simulink model "online_ups"  (R2024b)
settings: Solver=VariableStepAuto  StartTime=0.0  StopTime=0.2  RelTol=1e-3
libraries: spsIGBTDiodeLib x4, spsCurrentMeasurementLib x2, spsVoltageMeasurementLib x2, spsDCVoltageSourceLib x1, spsTriangleGeneratorLib x1, spsSeriesRLCBranchLib x1, sps_lib x1
settings Model: Creator=rushi  LastModifiedBy=rushi
settings DataIOCC: ReturnWorkspaceOutputs=off

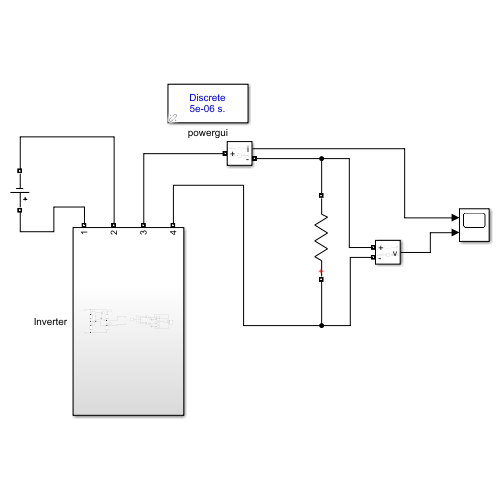
[thumbnail: Simulink's stored preview of the top-level diagram]
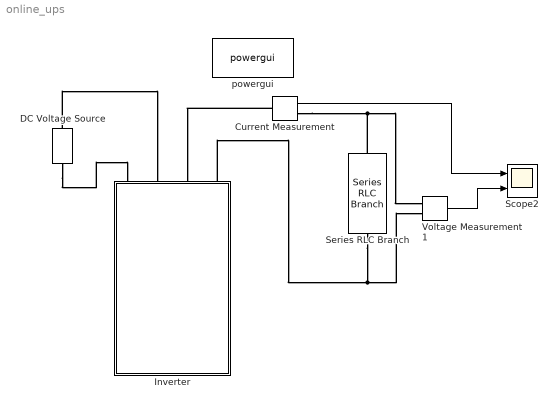
== system online_ups ==
  Current Measurement : spsCurrentMeasurementLib/Current Measurement  PhasorSimulation=off  OutputType=Complex  PSBequivalent=0
  DC Voltage Source : spsDCVoltageSourceLib/DC Voltage Source  Amplitude=100  Measurements=None
  Inverter : Subsystem
  Scope2 : Scope  NumInputPorts=2
  Series RLC Branch : spsSeriesRLCBranchLib/Series RLC Branch  LConnTagsString=__new0  RConnTagsString=__new0  BranchType=R  Resistance=1  Inductance=1e-3  SetiL0=off  InitialCurrent=0  Capacitance=1e-6  Setx0=off  InitialVoltage=0  Measurements=None
  Voltage Measurement1 : spsVoltageMeasurementLib/Voltage Measurement  PhasorSimulation=off  OutputType=Complex  PSBequivalent=0
  powergui : sps_lib/powergui  Priority=1  SimulationMode=Discrete  SampleTime=5e-6  frequency=60  Iterations=50  frequencyindice=0  Pbase=100e6  ErrMax=1e-4  UnitsV=kV  UnitsW=MW  buscounter=0  FunctionMessages=off  echomessages=off  EnableUseOfTLC=off  CurrentSourceSwitches=off  DisableSnubberDevices=off  DisableRonSwitches=off  DisableVfSwitches=off  DisplayEquations=off  AutomaticDiscreteSolvers=off  SolverType=Tustin/Backward Euler (TBE)  Interpol=off  ExternalGateDelay=off  methode=off  Ts=100  x0status=blocks  SPID=on  SwTol=0  HookPort=off  NonlinearTolerance=1e-4  nMaxIteration=100  ContinueOnMaxIteration=off  RestoreLinks=warning  ResistiveCurrentMeasurement=off  Frange=[0:2:500]  Ylog=off  Xlog=on  ShowGrid=off  save=off  variable=ZData  structure=0  ZoomFFT=off  StartTime=0.0  cycles=1  DisplayStyle=1  fundamental=60  FreqAxis=off  MaxFrequency=1000  frequencyindicesteady=1  RmsSteady=1  display=off
  wires:
  Voltage Measurement1/1 -> Scope2/2
  Current Measurement/1 -> Scope2/1
  connections:
  Series RLC Branch/RConn1 -- Current Measurement/RConn1 -- Voltage Measurement1/LConn1
  Series RLC Branch/LConn1 -- Inverter/LConn4 -- Voltage Measurement1/LConn2
  Current Measurement/LConn1 -- Inverter/LConn3
  DC Voltage Source/RConn1 -- Inverter/LConn1
  DC Voltage Source/LConn1 -- Inverter/LConn2

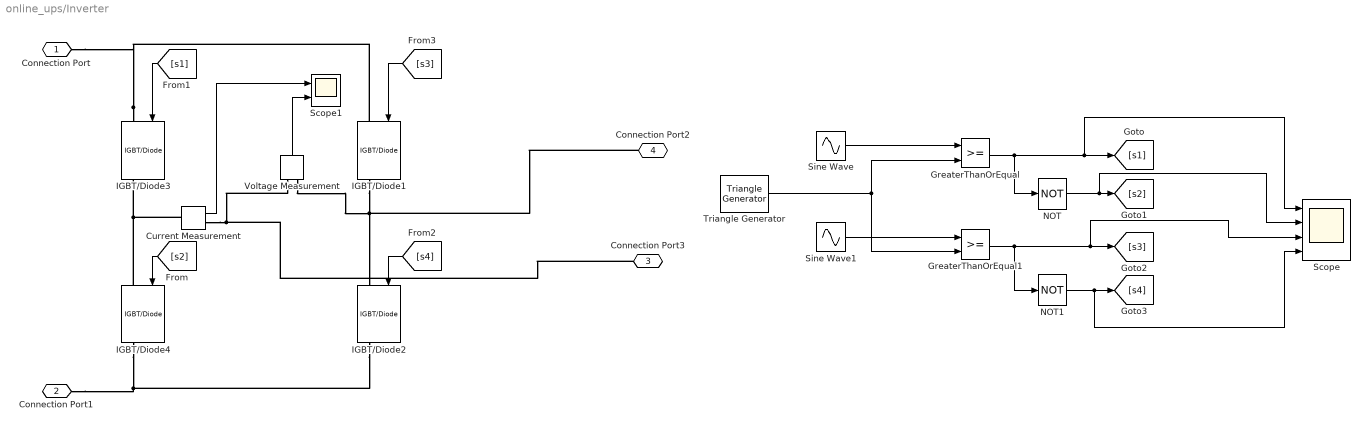
== system online_ups/Inverter ==
  Current Measurement : spsCurrentMeasurementLib/Current Measurement  PhasorSimulation=off  OutputType=Complex  PSBequivalent=0
  GreaterThanOrEqual : RelationalOperator  OutDataTypeStr=boolean  RndMeth=Simplest  InputSameDT=off
  GreaterThanOrEqual1 : RelationalOperator  OutDataTypeStr=boolean  RndMeth=Simplest  InputSameDT=off
  IGBT/Diode{1..4} (4 alike) : spsIGBTDiodeLib/IGBT//Diode  Ron=1e-3  Rs=1e5  Cs=inf  Measurements=on
  NOT : Logic  Operator=NOT  IconShape=distinctive  AllPortsSameDT=off  OutDataTypeStr=boolean
  NOT1 : Logic  Operator=NOT  IconShape=distinctive  AllPortsSameDT=off  OutDataTypeStr=boolean
  Scope : Scope  NumInputPorts=4
  Scope1 : Scope  NumInputPorts=2
  Sine Wave : Sin  Frequency=2*pi*50  SampleTime=0
  Sine Wave1 : Sin  Frequency=2*pi*50  Phase=pi  SampleTime=0
  Triangle Generator : spsTriangleGeneratorLib/Triangle Generator  Freq=1000  Phase=0  Ts=0
  Voltage Measurement : spsVoltageMeasurementLib/Voltage Measurement  PhasorSimulation=off  OutputType=Complex  PSBequivalent=0
  Connection Port : PMIOPort  Side=Left
  Connection Port1 : PMIOPort  Port=2  Side=Left
  Connection Port3 : PMIOPort  Port=3  Side=Left
  Connection Port2 : PMIOPort  Port=4  Side=Left
  wires:
  [s2] -> IGBT/Diode4/1
  [s1] -> IGBT/Diode3/1
  [s4] -> IGBT/Diode2/1
  Current Measurement/1 -> Scope1/1
  Voltage Measurement/1 -> Scope1/2
  [s3] -> IGBT/Diode1/1
  GreaterThanOrEqual/1 -> Scope/1, [s1], NOT/1
  GreaterThanOrEqual1/1 -> NOT1/1, Scope/3, [s3]
  Sine Wave1/1 -> GreaterThanOrEqual1/1
  Triangle Generator/1 -> GreaterThanOrEqual1/2, GreaterThanOrEqual/2
  Sine Wave/1 -> GreaterThanOrEqual/1
  NOT1/1 -> Scope/4, [s4]
  NOT/1 -> Scope/2, [s2]
  connections:
  IGBT/Diode4/RConn1 -- Connection Port1/RConn1 -- IGBT/Diode2/RConn1
  IGBT/Diode1/RConn1 -- Connection Port2/RConn1 -- IGBT/Diode2/LConn1 -- Voltage Measurement/LConn2
  Current Measurement/LConn1 -- IGBT/Diode4/LConn1 -- IGBT/Diode3/RConn1
  Voltage Measurement/LConn1 -- Connection Port3/RConn1 -- Current Measurement/RConn1
  IGBT/Diode3/LConn1 -- IGBT/Diode1/LConn1 -- Connection Port/RConn1
